simulink subsystem "SimscapeBatteryCircuitModel"  (R2024a)
settings: Solver=VariableStepAuto  StartTime=0.0  StopTime=10.0  RelTol=1e-3
values from neighbouring files (symbols this model uses):
  R = 0.05    [VehicleParameters.m]
  VRef = 600    [VehicleParameters.m]
libraries: fl_lib x4, nesl_utility x2
settings Model: Creator=44779  LastModifiedBy=44779

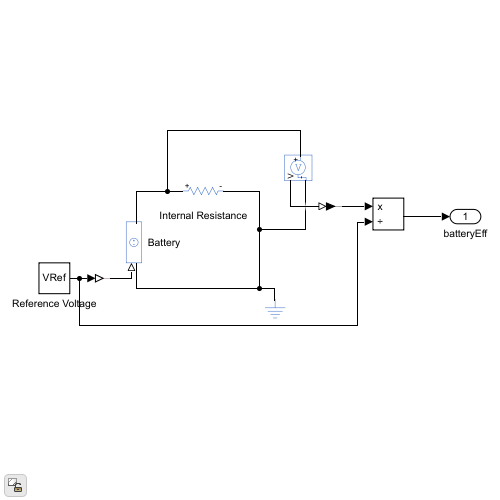
[thumbnail: Simulink's stored preview of the top-level diagram]
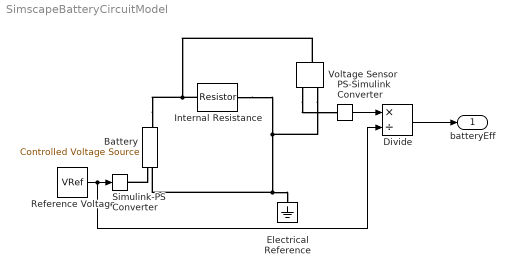
== system SimscapeBatteryCircuitModel ==
  Battery : fl_lib/Electrical/Electrical Sources/Controlled Voltage Source
  Divide : Product  Inputs=*/
  Electrical Reference : fl_lib/Electrical/Electrical Elements/Electrical Reference
  Internal Resistance : fl_lib/Electrical/Electrical Elements/Resistor  R=R Ohm  i_specify=off  i_priority=None  i=0 A  i_nominal_specify=off  i_nominal_value=1  i_nominal_unit=A  v_specify=off  v_priority=None  v=0 V  v_nominal_specify=off  v_nominal_value=1  v_nominal_unit=V
  PS-Simulink Converter : nesl_utility/PS-Simulink Converter  PhysicalDomain=network_engine_domain  SubClassName=ps_output  LeftPortType=input  RightPortType=output  PseudoPeriodic=off  Frequencies=[]  VectorFormat=inherit  Unit=inherit  AffineConversion=off
  Reference Voltage : Constant  Value=VRef
  Simulink-PS Converter : nesl_utility/Simulink-PS Converter  PhysicalDomain=network_engine_domain  SubClassName=ps_input  LeftPortType=input  RightPortType=output  PseudoPeriodic=off  Frequencies=[]  NoiseDistribution=none  NoiseParameters=[]  Unit=1  AffineConversion=off  FilteringAndDerivatives=provide  SimscapeFilterOrder=1  InputFilterTimeConstant=0.001  UdotUserProvided=0
  Voltage Sensor : fl_lib/Electrical/Electrical Sensors/Voltage Sensor
  batteryEff : Outport
  wires:
  PS-Simulink Converter/1 -> Divide/1
  Reference Voltage/1 -> Simulink-PS Converter/1, Divide/2
  Divide/1 -> batteryEff/1
  connections:
  Battery/LConn1 -- Internal Resistance/LConn1 -- Voltage Sensor/LConn1
  Internal Resistance/RConn1 -- Voltage Sensor/RConn2 -- Electrical Reference/LConn1 -- Battery/RConn2
  Voltage Sensor/RConn1 -- PS-Simulink Converter/LConn1
  Battery/RConn1 -- Simulink-PS Converter/RConn1
